simulink model "trace_track"  (R2016a)
settings: Solver=VariableStepAuto  StartTime=0.0  StopTime=100  RelTol=1e-3
undefined symbols (not defined in the file): A, B, C, D
settings Model: Creator=Gray  LastModifiedBy=Gray

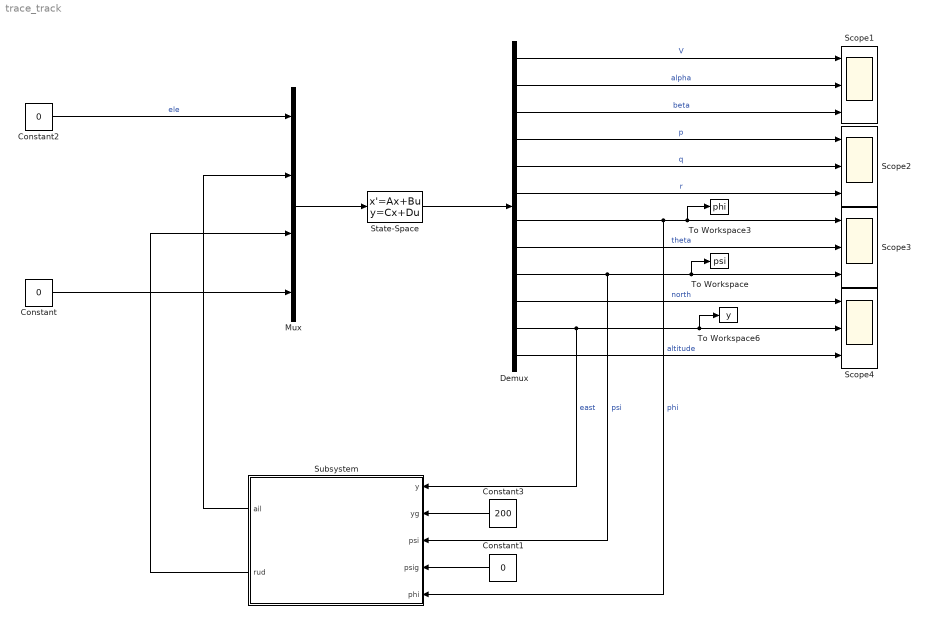
== system trace_track ==
  Constant : Constant  Value=0
  Constant1 : Constant  Value=0
  Constant2 : Constant  Value=0
  Constant3 : Constant  Value=200
  Demux : Demux  Outputs=12
  Mux : Mux
  Scope{1..4} (4 alike) : Scope  NumInputPorts=3
  State-Space : StateSpace  A=A  B=B  C=C  D=D  X0=[0 0 0 0 0 0 0 0 0 0 0 0]
  Subsystem : Subsystem
  To Workspace : ToWorkspace  VariableName=psi  SaveFormat=Timeseries  SampleTime=-1
  To Workspace3 : ToWorkspace  VariableName=phi  SaveFormat=Timeseries  SampleTime=-1
  To Workspace6 : ToWorkspace  VariableName=y  SaveFormat=Timeseries  SampleTime=-1
  wires:
  State-Space/1 -> Demux/1
  Mux/1 -> State-Space/1
  Demux/1 -> Scope1/1  "V"
  Demux/2 -> Scope1/2  "alpha"
  Demux/3 -> Scope1/3  "beta"
  Demux/4 -> Scope2/1  "p"
  Demux/5 -> Scope2/2  "q"
  Demux/6 -> Scope2/3  "r"
  Demux/7 -> Subsystem/5(phi), To Workspace3/1, Scope3/1  "phi"
  Demux/8 -> Scope3/2  "theta"
  Demux/9 -> Subsystem/3(psi), To Workspace/1, Scope3/3  "psi"
  Demux/10 -> Scope4/1  "north"
  Demux/11 -> Subsystem/1(y), To Workspace6/1, Scope4/2  "east"
  Demux/12 -> Scope4/3  "altitude"
  Constant/1 -> Mux/4
  Constant2/1 -> Mux/1  "ele"
  Constant1/1 -> Subsystem/4(psig)
  Subsystem/1(ail) -> Mux/2
  Subsystem/2(rud) -> Mux/3
  Constant3/1 -> Subsystem/2(yg)

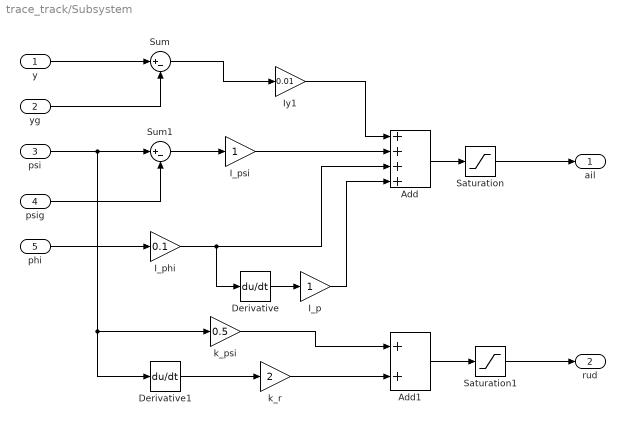
== system trace_track/Subsystem ==
  y : Inport
  yg : Inport  Port=2
  psi : Inport  Port=3
  psig : Inport  Port=4
  phi : Inport  Port=5
  Add : Sum  Inputs=++++
  Add1 : Sum
  Derivative : Derivative
  Derivative1 : Derivative
  I_p : Gain
  I_phi : Gain  Gain=0.1
  I_psi : Gain
  Iy1 : Gain  Gain=0.01
  Saturation : Saturate  UpperLimit=12  LowerLimit=-12
  Saturation1 : Saturate  UpperLimit=8  LowerLimit=-8
  Sum : Sum  Inputs=|+-
  Sum1 : Sum  Inputs=|+-
  k_psi : Gain  Gain=0.5
  k_r : Gain  Gain=2
  ail : Outport
  rud : Outport  Port=2
  wires:
  k_r/1 -> Add1/2
  k_psi/1 -> Add1/1
  Sum1/1 -> I_psi/1
  Add/1 -> Saturation/1
  Saturation/1 -> ail/1
  Add1/1 -> Saturation1/1
  Sum/1 -> Iy1/1
  Iy1/1 -> Add/1
  psi/1 -> Derivative1/1, k_psi/1, Sum1/1
  y/1 -> Sum/1
  psig/1 -> Sum1/2
  phi/1 -> I_phi/1
  I_phi/1 -> Derivative/1, Add/3
  Derivative/1 -> I_p/1
  Derivative1/1 -> k_r/1
  Saturation1/1 -> rud/1
  I_psi/1 -> Add/2
  I_p/1 -> Add/4
  yg/1 -> Sum/2
